simulink model "full_system"  (R2023b)
settings: Solver=VariableStepAuto  StartTime=0.0  StopTime=Tend  RelTol=1e-3
undefined symbols (not defined in the file): A, Af, B, beta_off_deg, beta_on_deg, C, Cd, control_case, D, f, g, G_rref, Ki_beta, Ki_r, Kp_beta, Kp_r, m, Mz_max, Mz_min, rho, rw, tf1, theta_front, Tmax_wheel, Tmin_wheel, tr
libraries: slpidlib x2
settings Model: Creator=GLORIA  LastModifiedBy=joseg
settings OptimizationCC: ReuseModelBlockBuffer=off

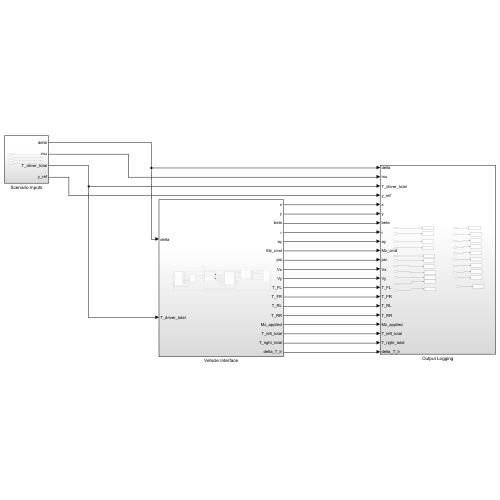
[thumbnail: Simulink's stored preview of the top-level diagram]
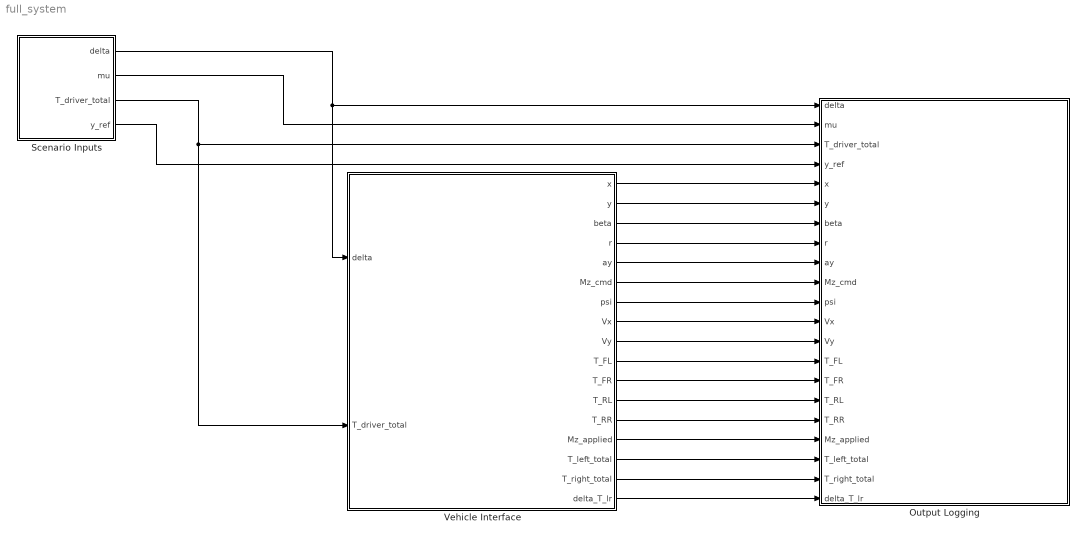
== system full_system ==
  Output Logging : Subsystem
  Scenario Inputs : Subsystem
  Vehicle Interface : Subsystem
  wires:
  Scenario Inputs/1(delta) -> Vehicle Interface/1(delta), Output Logging/1(delta)
  Scenario Inputs/2(mu) -> Output Logging/2(mu)
  Scenario Inputs/4(y_ref) -> Output Logging/4(y_ref)
  Vehicle Interface/1(x) -> Output Logging/5(x)
  Vehicle Interface/2(y) -> Output Logging/6(y)
  Vehicle Interface/3(beta) -> Output Logging/7(beta)
  Vehicle Interface/4(r) -> Output Logging/8(r)
  Vehicle Interface/5(ay) -> Output Logging/9(ay)
  Vehicle Interface/6(Mz_cmd) -> Output Logging/10(Mz_cmd)
  Vehicle Interface/7(psi) -> Output Logging/11(psi)
  Vehicle Interface/8(Vx) -> Output Logging/12(Vx)
  Vehicle Interface/9(Vy) -> Output Logging/13(Vy)
  Vehicle Interface/10(T_FL) -> Output Logging/14(T_FL)
  Vehicle Interface/11(T_FR) -> Output Logging/15(T_FR)
  Vehicle Interface/12(T_RL) -> Output Logging/16(T_RL)
  Vehicle Interface/13(T_RR) -> Output Logging/17(T_RR)
  Scenario Inputs/3(T_driver_total) -> Vehicle Interface/2(T_driver_total), Output Logging/3(T_driver_total)
  Vehicle Interface/14(Mz_applied) -> Output Logging/18(Mz_applied)
  Vehicle Interface/15(T_left_total) -> Output Logging/19(T_left_total)
  Vehicle Interface/16(T_right_total) -> Output Logging/20(T_right_total)
  Vehicle Interface/17(delta_T_lr) -> Output Logging/21(delta_T_lr)

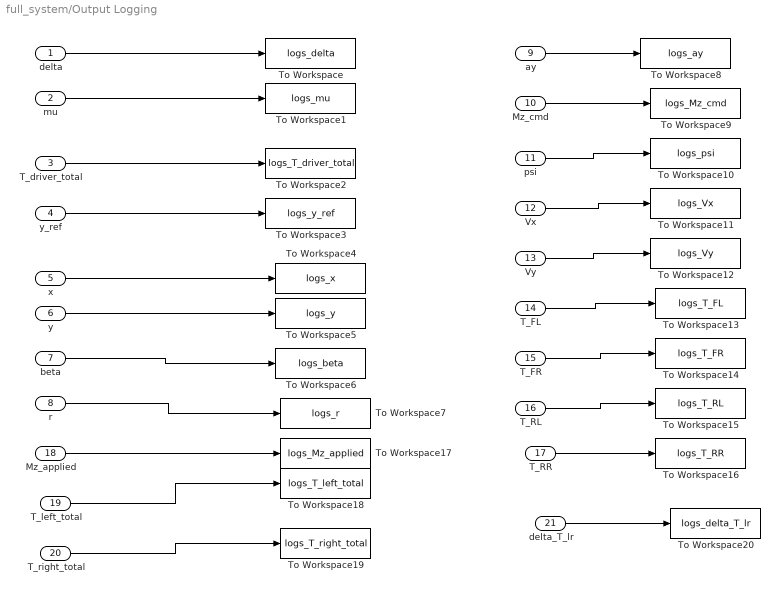
== system full_system/Output Logging ==
  delta : Inport
  mu : Inport  Port=2
  T_driver_total : Inport  Port=3
  y_ref : Inport  Port=4
  x : Inport  Port=5
  y : Inport  Port=6
  beta : Inport  Port=7
  r : Inport  Port=8
  ay : Inport  Port=9
  Mz_cmd : Inport  Port=10
  psi : Inport  Port=11
  Vx : Inport  Port=12
  Vy : Inport  Port=13
  T_FL : Inport  Port=14
  T_FR : Inport  Port=15
  T_RL : Inport  Port=16
  T_RR : Inport  Port=17
  Mz_applied : Inport  Port=18
  T_left_total : Inport  Port=19
  T_right_total : Inport  Port=20
  delta_T_lr : Inport  Port=21
  To Workspace : ToWorkspace  VariableName=logs_delta  SaveFormat=Timeseries  SampleTime=-1
  To Workspace1 : ToWorkspace  VariableName=logs_mu  SaveFormat=Timeseries  SampleTime=-1
  To Workspace10 : ToWorkspace  VariableName=logs_psi  SaveFormat=Timeseries  SampleTime=-1
  To Workspace11 : ToWorkspace  VariableName=logs_Vx  SaveFormat=Timeseries  SampleTime=-1
  To Workspace12 : ToWorkspace  VariableName=logs_Vy  SaveFormat=Timeseries  SampleTime=-1
  To Workspace13 : ToWorkspace  VariableName=logs_T_FL  SaveFormat=Timeseries  SampleTime=-1
  To Workspace14 : ToWorkspace  VariableName=logs_T_FR  SaveFormat=Timeseries  SampleTime=-1
  To Workspace15 : ToWorkspace  VariableName=logs_T_RL  SaveFormat=Timeseries  SampleTime=-1
  To Workspace16 : ToWorkspace  VariableName=logs_T_RR  SaveFormat=Timeseries  SampleTime=-1
  To Workspace17 : ToWorkspace  VariableName=logs_Mz_applied  SaveFormat=Timeseries  SampleTime=-1
  To Workspace18 : ToWorkspace  VariableName=logs_T_left_total  SaveFormat=Timeseries  SampleTime=-1
  To Workspace19 : ToWorkspace  VariableName=logs_T_right_total  SaveFormat=Timeseries  SampleTime=-1
  To Workspace2 : ToWorkspace  VariableName=logs_T_driver_total  SaveFormat=Timeseries  SampleTime=-1
  To Workspace20 : ToWorkspace  VariableName=logs_delta_T_lr  SaveFormat=Timeseries  SampleTime=-1
  To Workspace3 : ToWorkspace  VariableName=logs_y_ref  SaveFormat=Timeseries  SampleTime=-1
  To Workspace4 : ToWorkspace  VariableName=logs_x  SaveFormat=Timeseries  SampleTime=-1
  To Workspace5 : ToWorkspace  VariableName=logs_y  SaveFormat=Timeseries  SampleTime=-1
  To Workspace6 : ToWorkspace  VariableName=logs_beta  SaveFormat=Timeseries  SampleTime=-1
  To Workspace7 : ToWorkspace  VariableName=logs_r  SaveFormat=Timeseries  SampleTime=-1
  To Workspace8 : ToWorkspace  VariableName=logs_ay  SaveFormat=Timeseries  SampleTime=-1
  To Workspace9 : ToWorkspace  VariableName=logs_Mz_cmd  SaveFormat=Timeseries  SampleTime=-1
  wires:
  delta/1 -> To Workspace/1
  mu/1 -> To Workspace1/1
  T_driver_total/1 -> To Workspace2/1
  y_ref/1 -> To Workspace3/1
  x/1 -> To Workspace4/1
  y/1 -> To Workspace5/1
  beta/1 -> To Workspace6/1
  r/1 -> To Workspace7/1
  ay/1 -> To Workspace8/1
  Mz_cmd/1 -> To Workspace9/1
  psi/1 -> To Workspace10/1
  Vx/1 -> To Workspace11/1
  Vy/1 -> To Workspace12/1
  T_FL/1 -> To Workspace13/1
  T_FR/1 -> To Workspace14/1
  T_RL/1 -> To Workspace15/1
  T_RR/1 -> To Workspace16/1
  Mz_applied/1 -> To Workspace17/1
  delta_T_lr/1 -> To Workspace20/1
  T_left_total/1 -> To Workspace18/1
  T_right_total/1 -> To Workspace19/1

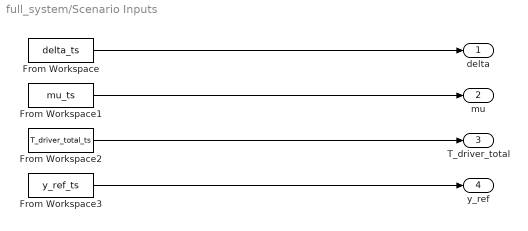
== system full_system/Scenario Inputs ==
  From Workspace : FromWorkspace  VariableName=delta_ts
  From Workspace1 : FromWorkspace  VariableName=mu_ts
  From Workspace2 : FromWorkspace  VariableName=T_driver_total_ts
  From Workspace3 : FromWorkspace  VariableName=y_ref_ts
  delta : Outport
  mu : Outport  Port=2
  T_driver_total : Outport  Port=3
  y_ref : Outport  Port=4
  wires:
  From Workspace/1 -> delta/1
  From Workspace1/1 -> mu/1
  From Workspace2/1 -> T_driver_total/1
  From Workspace3/1 -> y_ref/1

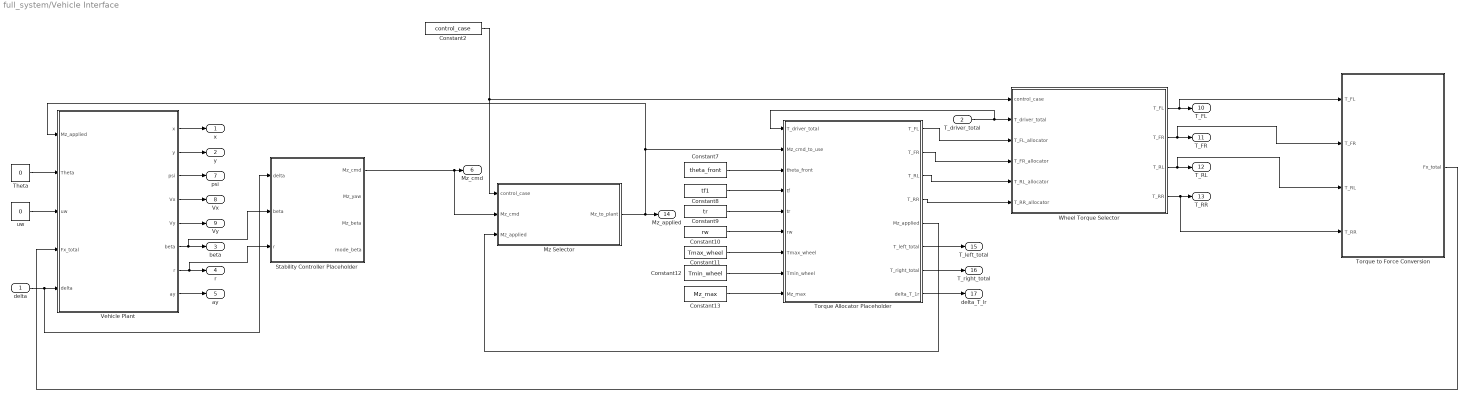
== system full_system/Vehicle Interface ==
  delta : Inport
  T_driver_total : Inport  Port=2
  Constant10 : Constant  Value=rw
  Constant11 : Constant  Value=Tmax_wheel
  Constant12 : Constant  Value=Tmin_wheel
  Constant13 : Constant  Value=Mz_max
  Constant2 : Constant  Value=control_case
  Constant7 : Constant  Value=theta_front
  Constant8 : Constant  Value=tf1
  Constant9 : Constant  Value=tr
  Mz Selector : Subsystem
  Stability Controller Placeholder : Subsystem
  Theta : Constant  Value=0
  Torque Allocator Placeholder : Subsystem
  Torque to Force Conversion : Subsystem
  Vehicle Plant : Subsystem
  Wheel Torque Selector : Subsystem
  uw : Constant  Value=0
  x : Outport
  y : Outport  Port=2
  beta : Outport  Port=3
  r : Outport  Port=4
  ay : Outport  Port=5
  Mz_cmd : Outport  Port=6
  psi : Outport  Port=7
  Vx : Outport  Port=8
  Vy : Outport  Port=9
  T_FL : Outport  Port=10
  T_FR : Outport  Port=11
  T_RL : Outport  Port=12
  T_RR : Outport  Port=13
  Mz_applied : Outport  Port=14
  T_left_total : Outport  Port=15
  T_right_total : Outport  Port=16
  delta_T_lr : Outport  Port=17
  wires:
  Theta/1 -> Vehicle Plant/2(Theta)
  uw/1 -> Vehicle Plant/3(uw)
  Vehicle Plant/1(x) -> x/1
  Vehicle Plant/2(y) -> y/1
  Vehicle Plant/3(psi) -> psi/1
  Vehicle Plant/4(Vx) -> Vx/1
  Vehicle Plant/5(Vy) -> Vy/1
  Vehicle Plant/6(beta) -> beta/1, Stability Controller Placeholder/2(beta)
  Vehicle Plant/7(r) -> r/1, Stability Controller Placeholder/3(r)
  Vehicle Plant/8(ay) -> ay/1
  T_driver_total/1 -> Torque Allocator Placeholder/1(T_driver_total), Wheel Torque Selector/2(T_driver_total)
  Torque to Force Conversion/1(Fx_total) -> Vehicle Plant/4(Fx_total)
  delta/1 -> Vehicle Plant/5(delta), Stability Controller Placeholder/1(delta)
  Stability Controller Placeholder/1(Mz_cmd) -> Mz Selector/2(Mz_cmd), Mz_cmd/1
  Mz Selector/1(Mz_to_plant) -> Mz_applied/1, Torque Allocator Placeholder/2(Mz_cmd_to_use), Vehicle Plant/1(Mz_applied)
  Wheel Torque Selector/1(T_FL) -> T_FL/1, Torque to Force Conversion/1(T_FL)
  Wheel Torque Selector/2(T_FR) -> Torque to Force Conversion/2(T_FR), T_FR/1
  Wheel Torque Selector/3(T_RL) -> T_RL/1, Torque to Force Conversion/3(T_RL)
  Wheel Torque Selector/4(T_RR) -> Torque to Force Conversion/4(T_RR), T_RR/1
  Torque Allocator Placeholder/1(T_FL) -> Wheel Torque Selector/3(T_FL_allocator)
  Torque Allocator Placeholder/2(T_FR) -> Wheel Torque Selector/4(T_FR_allocator)
  Torque Allocator Placeholder/3(T_RL) -> Wheel Torque Selector/5(T_RL_allocator)
  Torque Allocator Placeholder/4(T_RR) -> Wheel Torque Selector/6(T_RR_allocator)
  Torque Allocator Placeholder/5(Mz_applied) -> Mz Selector/3(Mz_applied)
  Constant2/1 -> Mz Selector/1(control_case), Wheel Torque Selector/1(control_case)
  Torque Allocator Placeholder/6(T_left_total) -> T_left_total/1
  Torque Allocator Placeholder/8(delta_T_1r) -> delta_T_lr/1
  Torque Allocator Placeholder/7(T_right_total) -> T_right_total/1
  Constant7/1 -> Torque Allocator Placeholder/3(theta_front)
  Constant8/1 -> Torque Allocator Placeholder/4(tf)
  Constant9/1 -> Torque Allocator Placeholder/5(tr)
  Constant10/1 -> Torque Allocator Placeholder/6(rw)
  Constant11/1 -> Torque Allocator Placeholder/7(Tmax_wheel)
  Constant12/1 -> Torque Allocator Placeholder/8(Tmin_wheel)
  Constant13/1 -> Torque Allocator Placeholder/9(Mz_max)

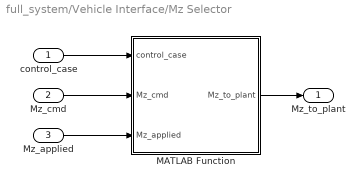
== system full_system/Vehicle Interface/Mz Selector ==
  control_case : Inport
  Mz_cmd : Inport  Port=2
  Mz_applied : Inport  Port=3
  MATLAB Function : MATLAB Function  TreatAsAtomicUnit=on
  Mz_to_plant : Outport
  wires:
  MATLAB Function/1(Mz_to_plant) -> Mz_to_plant/1
  Mz_cmd/1 -> MATLAB Function/2(Mz_cmd)
  Mz_applied/1 -> MATLAB Function/3(Mz_applied)
  control_case/1 -> MATLAB Function/1(control_case)

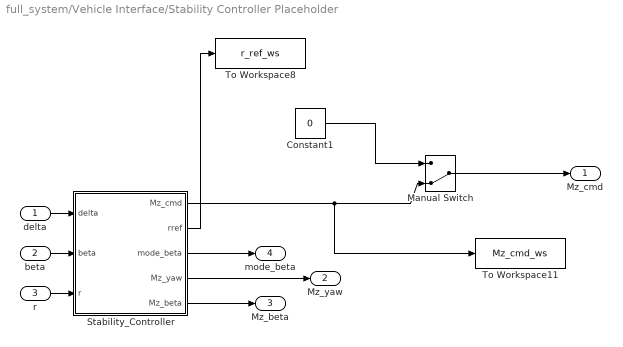
== system full_system/Vehicle Interface/Stability Controller Placeholder ==
  delta : Inport
  beta : Inport  Port=2
  r : Inport  Port=3
  Constant1 : Constant  Value=0
  Manual Switch : ManualSwitch  CurrentSetting=0
  Stability_Controller : Subsystem
  To Workspace11 : ToWorkspace  VariableName=Mz_cmd_ws  SaveFormat=Structure With Time  SampleTime=-1
      settings: Save2DSignal=2-D array (concatenate along first dimension)
  To Workspace8 : ToWorkspace  VariableName=r_ref_ws  SaveFormat=Structure With Time  SampleTime=-1
      settings: Save2DSignal=2-D array (concatenate along first dimension)
  Mz_cmd : Outport
  Mz_yaw : Outport  Port=2
  Mz_beta : Outport  Port=3
  mode_beta : Outport  Port=4
  wires:
  Stability_Controller/1(Mz_cmd) -> To Workspace11/1, Manual Switch/2
  Stability_Controller/2(rref) -> To Workspace8/1
  Constant1/1 -> Manual Switch/1
  delta/1 -> Stability_Controller/1(delta)
  beta/1 -> Stability_Controller/2(beta)
  r/1 -> Stability_Controller/3(r)
  Stability_Controller/3(mode_beta) -> mode_beta/1
  Manual Switch/1 -> Mz_cmd/1
  Stability_Controller/5(Mz_beta) -> Mz_beta/1
  Stability_Controller/4(Mz_yaw) -> Mz_yaw/1

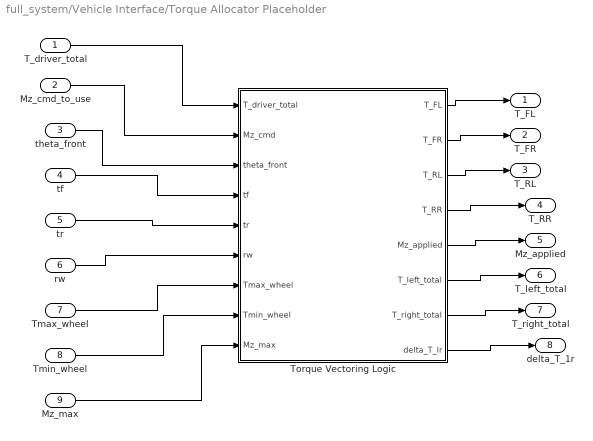
== system full_system/Vehicle Interface/Torque Allocator Placeholder ==
  T_driver_total : Inport
  Mz_cmd_to_use : Inport  Port=2
  theta_front : Inport  Port=3
  tf : Inport  Port=4
  tr : Inport  Port=5
  rw : Inport  Port=6
  Tmax_wheel : Inport  Port=7
  Tmin_wheel : Inport  Port=8
  Mz_max : Inport  Port=9
  Torque Vectoring Logic : MATLAB Function  TreatAsAtomicUnit=on
  T_FL : Outport
  T_FR : Outport  Port=2
  T_RL : Outport  Port=3
  T_RR : Outport  Port=4
  Mz_applied : Outport  Port=5
  T_left_total : Outport  Port=6
  T_right_total : Outport  Port=7
  delta_T_1r : Outport  Port=8
  wires:
  theta_front/1 -> Torque Vectoring Logic/3(theta_front)
  Tmax_wheel/1 -> Torque Vectoring Logic/7(Tmax_wheel)
  tr/1 -> Torque Vectoring Logic/5(tr)
  Mz_cmd_to_use/1 -> Torque Vectoring Logic/2(Mz_cmd)
  Tmin_wheel/1 -> Torque Vectoring Logic/8(Tmin_wheel)
  Mz_max/1 -> Torque Vectoring Logic/9(Mz_max)
  tf/1 -> Torque Vectoring Logic/4(tf)
  rw/1 -> Torque Vectoring Logic/6(rw)
  Torque Vectoring Logic/1(T_FL) -> T_FL/1
  Torque Vectoring Logic/2(T_FR) -> T_FR/1
  Torque Vectoring Logic/3(T_RL) -> T_RL/1
  Torque Vectoring Logic/4(T_RR) -> T_RR/1
  Torque Vectoring Logic/5(Mz_applied) -> Mz_applied/1
  Torque Vectoring Logic/6(T_left_total) -> T_left_total/1
  Torque Vectoring Logic/7(T_right_total) -> T_right_total/1
  Torque Vectoring Logic/8(delta_T_lr) -> delta_T_1r/1
  T_driver_total/1 -> Torque Vectoring Logic/1(T_driver_total)

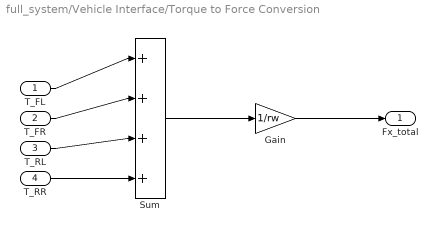
== system full_system/Vehicle Interface/Torque to Force Conversion ==
  T_FL : Inport
  T_FR : Inport  Port=2
  T_RL : Inport  Port=3
  T_RR : Inport  Port=4
  Gain : Gain  Gain=1/rw
  Sum : Sum  Inputs=|++++
  Fx_total : Outport
  wires:
  Gain/1 -> Fx_total/1
  T_FL/1 -> Sum/1
  T_FR/1 -> Sum/2
  T_RL/1 -> Sum/3
  T_RR/1 -> Sum/4
  Sum/1 -> Gain/1

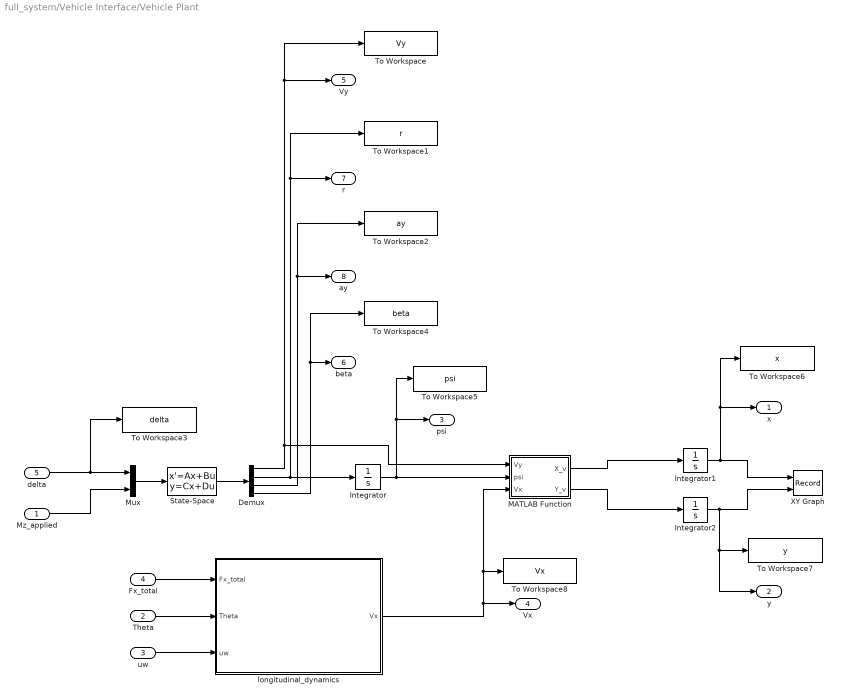
== system full_system/Vehicle Interface/Vehicle Plant ==
  Mz_applied : Inport
  Theta : Inport  Port=2
  uw : Inport  Port=3
  Fx_total : Inport  Port=4
  delta : Inport  Port=5
  Demux : Demux
  Integrator : Integrator
  Integrator1 : Integrator
  Integrator2 : Integrator
  MATLAB Function : MATLAB Function  TreatAsAtomicUnit=on
  Mux : Mux  Inputs=2
  State-Space : StateSpace  A=A  B=B  C=C  D=D  InitialCondition=[0;0]
  To Workspace : ToWorkspace  VariableName=Vy  SampleTime=-1
      settings: Save2DSignal=2-D array (concatenate along first dimension)
  To Workspace1 : ToWorkspace  VariableName=r  SampleTime=-1
      settings: Save2DSignal=2-D array (concatenate along first dimension)
  To Workspace2 : ToWorkspace  VariableName=ay  SampleTime=-1
      settings: Save2DSignal=2-D array (concatenate along first dimension)
  To Workspace3 : ToWorkspace  VariableName=delta  SampleTime=-1
      settings: Save2DSignal=2-D array (concatenate along first dimension)
  To Workspace4 : ToWorkspace  VariableName=beta  SampleTime=-1
      settings: Save2DSignal=2-D array (concatenate along first dimension)
  To Workspace5 : ToWorkspace  VariableName=psi  SampleTime=-1
      settings: Save2DSignal=2-D array (concatenate along first dimension)
  To Workspace6 : ToWorkspace  VariableName=x  SampleTime=-1
      settings: Save2DSignal=2-D array (concatenate along first dimension)
  To Workspace7 : ToWorkspace  VariableName=y  SampleTime=-1
      settings: Save2DSignal=2-D array (concatenate along first dimension)
  To Workspace8 : ToWorkspace  VariableName=Vx  SampleTime=-1
      settings: Save2DSignal=2-D array (concatenate along first dimension)
  XY Graph : Record  FileSettingsInternal="{\"entries\":[{\"content\":{\"excelSettings\":{\"content\":{},\"type\":\"Streamout.ExcelSettings\"}},\"type\":\"Streamout.FileSettingStorage\",\"uuid\":\"\"}],\"packageUris\":[\"http:\\/\\/schema.mathworks.com\\/mf0\\/streamout_blocks\\/R2020a\"],\"version\":\"1.0\"}"  Layout=[1 1]  SignalsInternal="{\"entries\":[{\"content\":{\"signals\":[{\"content\":{\"blockPath\":[],\"dimensions\":[1],\"domain\":\"\",\"lineColor\":\"#ff6929\",\"port\":1,\"signalID\":1,\"signalName\":\"Integrator1\"},\"type\":\"RecordBlkView.Signal\",\"uuid\":\"\"},{\"content\":{\"blockPath\":[],\"dimensions\":[1],\"domain\":\"\",\"lineColor\":\"#139fff\",\"plots\":[ 1 ],\"port\":2,\"signalID\":2,\"signalName\":\"Integrator2\"},\"type\":\"RecordBlkView.Signal\",\"uuid\":\"\"}]},\"type\":\"RecordBlkView.InputSignals\",\"uuid\":\"\"}],\"packageUris\":[\"http:\\/\\/schema.mathworks.com\\/mf0\\/streamout_blocks\\/R2020a\"],\"version\":\"1.0\"}"  VisualizationBindings="{\"xyplotplugin\":{\"info\":[{\"series\":[{\"bindingParametersList\":[{\"parameter\":\"Y-Axis\",\"signalID\":2,\"signalName\":\"Integrator2\"}],\"seriesID\":0}],\"subplotID\":1}]}}"  CompatibilityTag=XY
  longitudinal_dynamics : Subsystem
  x : Outport
  y : Outport  Port=2
  psi : Outport  Port=3
  Vx : Outport  Port=4
  Vy : Outport  Port=5
  beta : Outport  Port=6
  r : Outport  Port=7
  ay : Outport  Port=8
  wires:
  Integrator/1 -> psi/1, To Workspace5/1, MATLAB Function/2(psi)
  Demux/3 -> To Workspace2/1, ay/1
  Demux/4 -> To Workspace4/1, beta/1
  Integrator2/1 -> y/1, To Workspace7/1, XY Graph/2
  Integrator1/1 -> x/1, To Workspace6/1, XY Graph/1
  Demux/1 -> To Workspace/1, Vy/1, MATLAB Function/1(Vy)
  Theta/1 -> longitudinal_dynamics/2(Theta)
  MATLAB Function/2(Y_v) -> Integrator2/1
  Mux/1 -> State-Space/1
  MATLAB Function/1(X_v) -> Integrator1/1
  longitudinal_dynamics/1(Vx) -> MATLAB Function/3(Vx), To Workspace8/1, Vx/1
  State-Space/1 -> Demux/1
  uw/1 -> longitudinal_dynamics/3(uw)
  Mz_applied/1 -> Mux/2
  Demux/2 -> To Workspace1/1, r/1, Integrator/1
  Fx_total/1 -> longitudinal_dynamics/1(Fx_total)
  delta/1 -> Mux/1, To Workspace3/1

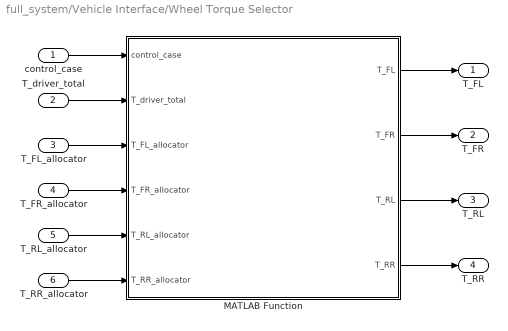
== system full_system/Vehicle Interface/Wheel Torque Selector ==
  control_case : Inport
  T_driver_total : Inport  Port=2
  T_FL_allocator : Inport  Port=3
  T_FR_allocator : Inport  Port=4
  T_RL_allocator : Inport  Port=5
  T_RR_allocator : Inport  Port=6
  MATLAB Function : MATLAB Function  TreatAsAtomicUnit=on
  T_FL : Outport
  T_FR : Outport  Port=2
  T_RL : Outport  Port=3
  T_RR : Outport  Port=4
  wires:
  MATLAB Function/1(T_FL) -> T_FL/1
  MATLAB Function/2(T_FR) -> T_FR/1
  MATLAB Function/3(T_RL) -> T_RL/1
  MATLAB Function/4(T_RR) -> T_RR/1
  control_case/1 -> MATLAB Function/1(control_case)
  T_driver_total/1 -> MATLAB Function/2(T_driver_total)
  T_FL_allocator/1 -> MATLAB Function/3(T_FL_allocator)
  T_RL_allocator/1 -> MATLAB Function/5(T_RL_allocator)
  T_FR_allocator/1 -> MATLAB Function/4(T_FR_allocator)
  T_RR_allocator/1 -> MATLAB Function/6(T_RR_allocator)

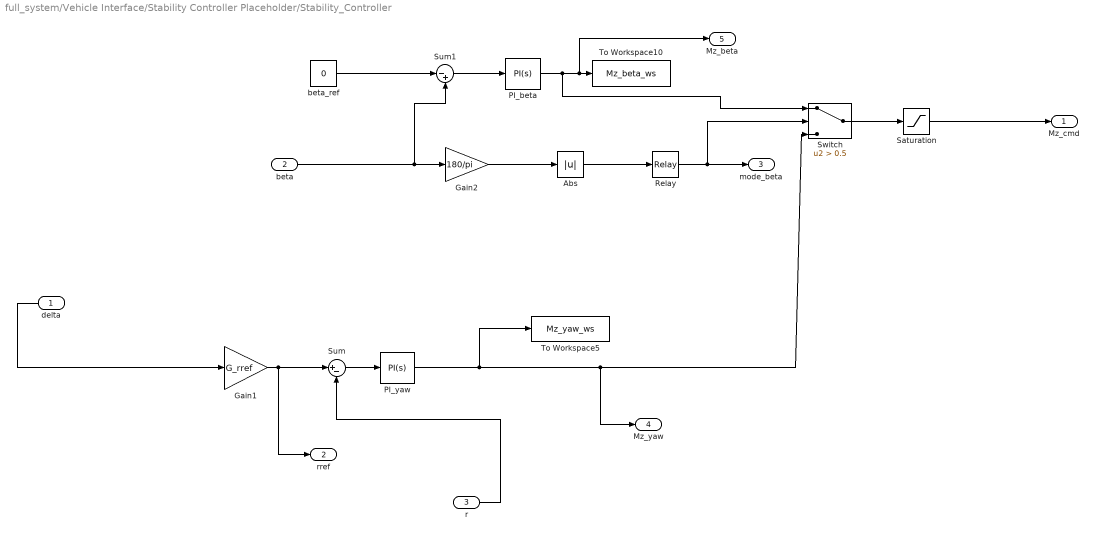
== system full_system/Vehicle Interface/Stability Controller Placeholder/Stability_Controller ==
  delta : Inport
  beta : Inport  Port=2
  r : Inport  Port=3
  Abs : Abs  SaturateOnIntegerOverflow=off
  Gain1 : Gain  Gain=G_rref
  Gain2 : Gain  Gain=180/pi
  PI_beta : slpidlib/PID Controller  Controller=PI  Form=Parallel  TimeDomain=Continuous-time  UseExternalTs=off  SampleTime=-1  IntegratorMethod=Forward Euler  FilterMethod=Forward Euler  ControllerParametersSource=internal  P=Kp_beta  I=Ki_beta  UseKiTs=off  D=0  N=100  UseFilter=on  TunerSelectOption=Transfer Function Based (PID Tuner App)  InitialConditionSource=internal  InitialConditionForIntegrator=0  InitialConditionForFilter=0  DifferentiatorICPrevScaledInput=0  ExternalReset=none  TrackingMode=off  Kt=1  LimitOutput=off  SatLimitsSource=internal  UpperSaturationLimit=inf  LowerSaturationLimit=-inf  LinearizeAsGain=on  AntiWindupMode=none  Kb=1  LimitIntegrator=off  UpperIntegratorSaturationLimit=inf  LowerIntegratorSaturationLimit=-inf  POutMin=[]  POutMax=[]  IOutMin=[]  IOutMax=[]  DOutMin=[]  DOutMax=[]  NOutMin=[]  NOutMax=[]  SumOutMin=[]  SumOutMax=[]  SaturationOutMin=[]  SaturationOutMax=[]  PParamMin=[]  PParamMax=[]  IParamMin=[]  IParamMax=[]  DParamMin=[]  DParamMax=[]  NParamMin=[]  NParamMax=[]  KbParamMin=[]  KbParamMax=[]  KtParamMin=[]  KtParamMax=[]  KbOutMin=[]  KbOutMax=[]  KtOutMin=[]  KtOutMax=[]  IntegratorOutMin=[]  IntegratorOutMax=[]  FilterOutMin=[]  FilterOutMax=[]  SumI1OutMin=[]  SumI1OutMax=[]  SumI2OutMin=[]  SumI2OutMax=[]  SumI3OutMin=[]  SumI3OutMax=[]  SumI4OutMin=[]  SumI4OutMax=[]  SumDOutMin=[]  SumDOutMax=[]  DifferentiatorOutMin=[]  DifferentiatorOutMax=[]  FilterDiffOutCoefMin=[]  FilterDiffOutCoefMax=[]  ReciprocalOutMin=[]  ReciprocalOutMax=[]  SumDenOutMin=[]  SumDenOutMax=[]  SumNumOutMin=[]  SumNumOutMax=[]  DivideOutMin=[]  DivideOutMax=[]  UdiffTsProdOutMin=[]  UdiffTsProdOutMax=[]  NTsProdOutMin=[]  NTsProdOutMax=[]  UintegralTsProdOutMin=[]  UintegralTsProdOutMax=[]  UngainTsProdOutMin=[]  UngainTsProdOutMax=[]  ClampingZeroOutDataTypeStr=Inherit: Inherit via back propagation  ClampingZeroOutMin=[]  ClampingZeroOutMax=[]  FilterDenConstantOutDataTypeStr=Inherit: Inherit via back propagation  FilterDenConstantOutMin=[]  FilterDenConstantOutMax=[]  PCopyOutDataTypeStr=Inherit: Inherit via back propagation  PCopyOutMin=[]  PCopyOutMax=[]  NCopyOutDataTypeStr=Inherit: Inherit via back propagation  NCopyOutMin=[]  NCopyOutMax=[]  IntegratorContinuousStateAttributes=''  IntegratorStateMustResolveToSignalObject=off  IntegratorRTWStateStorageClass=Auto  FilterContinuousStateAttributes=''  FilterStateMustResolveToSignalObject=off  FilterRTWStateStorageClass=Auto  ParallelPVariant=InternalParameters  IdealPVariant=Disabled  IVariant=InternalParameters  DVariant=Disabled  IntegratorVariant=Continuous  SatVariant=Disabled  AWVariant=Passthrough  PCopyVariant=Disabled  TRVariant=Disabled  FdbkBlocksVariant=Forward  IdealPFdbkVariant=Disabled  SatFdbkVariant=Disabled  DerivativeFilterVariant=Disabled  NVariant=Disabled  NCopyVariant=Disabled_SignalSpec  FilterICVariant=Disabled  IntegratorICVariant=InternalICs  ExternalResetVariant=Disabled  TRSumVariant=Passthrough  SumFdbkVariant=Disabled  SumVariant=Sum_PI  TsampFilterVariant=InternalTs  TsampNgainVariant=Passthrough  TsampIntegralVariant=Disabled_SignalSpec  ExternalSaturationOutDataTypeStr=Inherit: Same as second input
  PI_yaw : slpidlib/PID Controller  Controller=PI  Form=Parallel  TimeDomain=Continuous-time  UseExternalTs=off  SampleTime=-1  IntegratorMethod=Forward Euler  FilterMethod=Forward Euler  ControllerParametersSource=internal  P=Kp_r  I=Ki_r  UseKiTs=off  D=0  N=100  UseFilter=on  TunerSelectOption=Transfer Function Based (PID Tuner App)  InitialConditionSource=internal  InitialConditionForIntegrator=0  InitialConditionForFilter=0  DifferentiatorICPrevScaledInput=0  ExternalReset=none  TrackingMode=off  Kt=1  LimitOutput=off  SatLimitsSource=internal  UpperSaturationLimit=inf  LowerSaturationLimit=-inf  LinearizeAsGain=on  AntiWindupMode=none  Kb=1  LimitIntegrator=off  UpperIntegratorSaturationLimit=inf  LowerIntegratorSaturationLimit=-inf  POutMin=[]  POutMax=[]  IOutMin=[]  IOutMax=[]  DOutMin=[]  DOutMax=[]  NOutMin=[]  NOutMax=[]  SumOutMin=[]  SumOutMax=[]  SaturationOutMin=[]  SaturationOutMax=[]  PParamMin=[]  PParamMax=[]  IParamMin=[]  IParamMax=[]  DParamMin=[]  DParamMax=[]  NParamMin=[]  NParamMax=[]  KbParamMin=[]  KbParamMax=[]  KtParamMin=[]  KtParamMax=[]  KbOutMin=[]  KbOutMax=[]  KtOutMin=[]  KtOutMax=[]  IntegratorOutMin=[]  IntegratorOutMax=[]  FilterOutMin=[]  FilterOutMax=[]  SumI1OutMin=[]  SumI1OutMax=[]  SumI2OutMin=[]  SumI2OutMax=[]  SumI3OutMin=[]  SumI3OutMax=[]  SumI4OutMin=[]  SumI4OutMax=[]  SumDOutMin=[]  SumDOutMax=[]  DifferentiatorOutMin=[]  DifferentiatorOutMax=[]  FilterDiffOutCoefMin=[]  FilterDiffOutCoefMax=[]  ReciprocalOutMin=[]  ReciprocalOutMax=[]  SumDenOutMin=[]  SumDenOutMax=[]  SumNumOutMin=[]  SumNumOutMax=[]  DivideOutMin=[]  DivideOutMax=[]  UdiffTsProdOutMin=[]  UdiffTsProdOutMax=[]  NTsProdOutMin=[]  NTsProdOutMax=[]  UintegralTsProdOutMin=[]  UintegralTsProdOutMax=[]  UngainTsProdOutMin=[]  UngainTsProdOutMax=[]  ClampingZeroOutDataTypeStr=Inherit: Inherit via back propagation  ClampingZeroOutMin=[]  ClampingZeroOutMax=[]  FilterDenConstantOutDataTypeStr=Inherit: Inherit via back propagation  FilterDenConstantOutMin=[]  FilterDenConstantOutMax=[]  PCopyOutDataTypeStr=Inherit: Inherit via back propagation  PCopyOutMin=[]  PCopyOutMax=[]  NCopyOutDataTypeStr=Inherit: Inherit via back propagation  NCopyOutMin=[]  NCopyOutMax=[]  IntegratorContinuousStateAttributes=''  IntegratorStateMustResolveToSignalObject=off  IntegratorRTWStateStorageClass=Auto  FilterContinuousStateAttributes=''  FilterStateMustResolveToSignalObject=off  FilterRTWStateStorageClass=Auto  ParallelPVariant=InternalParameters  IdealPVariant=Disabled  IVariant=InternalParameters  DVariant=Disabled  IntegratorVariant=Continuous  SatVariant=Disabled  AWVariant=Passthrough  PCopyVariant=Disabled  TRVariant=Disabled  FdbkBlocksVariant=Forward  IdealPFdbkVariant=Disabled  SatFdbkVariant=Disabled  DerivativeFilterVariant=Disabled  NVariant=Disabled  NCopyVariant=Disabled_SignalSpec  FilterICVariant=Disabled  IntegratorICVariant=InternalICs  ExternalResetVariant=Disabled  TRSumVariant=Passthrough  SumFdbkVariant=Disabled  SumVariant=Sum_PI  TsampFilterVariant=InternalTs  TsampNgainVariant=Passthrough  TsampIntegralVariant=Disabled_SignalSpec  ExternalSaturationOutDataTypeStr=Inherit: Same as second input
  Relay : Relay  OnSwitchValue=beta_on_deg  OffSwitchValue=beta_off_deg
  Saturation : Saturate  UpperLimit=Mz_max  LowerLimit=Mz_min
  Sum : Sum  Inputs=|+-
  Sum1 : Sum  Inputs=|-+
  Switch : Switch  Criteria=u2 > Threshold  Threshold=0.5  SaturateOnIntegerOverflow=off  InputSameDT=off
  To Workspace10 : ToWorkspace  VariableName=Mz_beta_ws  SaveFormat=Structure With Time  SampleTime=-1
      settings: Save2DSignal=2-D array (concatenate along first dimension)
  To Workspace5 : ToWorkspace  VariableName=Mz_yaw_ws  SaveFormat=Structure With Time  SampleTime=-1
      settings: Save2DSignal=2-D array (concatenate along first dimension)
  beta_ref : Constant  Value=0
  Mz_cmd : Outport
  rref : Outport  Port=2
  mode_beta : Outport  Port=3
  Mz_yaw : Outport  Port=4
  Mz_beta : Outport  Port=5
  wires:
  beta_ref/1 -> Sum1/1
  Abs/1 -> Relay/1
  PI_beta/1 -> Switch/1, Mz_beta/1, To Workspace10/1
  beta/1 -> Sum1/2, Gain2/1
  PI_yaw/1 -> To Workspace5/1, Mz_yaw/1, Switch/3
  Gain2/1 -> Abs/1
  Sum/1 -> PI_yaw/1
  Sum1/1 -> PI_beta/1
  Gain1/1 -> rref/1, Sum/1
  delta/1 -> Gain1/1
  r/1 -> Sum/2
  Switch/1 -> Saturation/1
  Saturation/1 -> Mz_cmd/1
  Relay/1 -> Switch/2, mode_beta/1

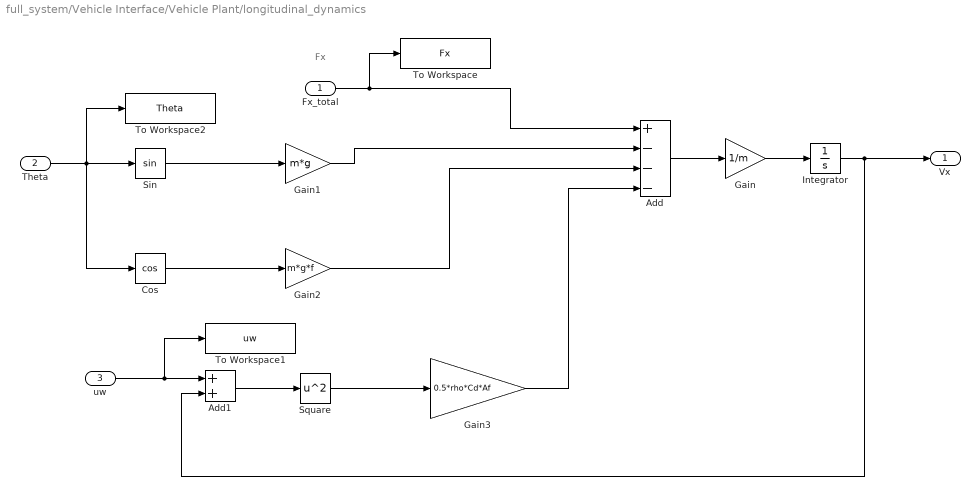
== system full_system/Vehicle Interface/Vehicle Plant/longitudinal_dynamics ==
  note: Fx
  Fx_total : Inport
  Theta : Inport  Port=2
  uw : Inport  Port=3
  Add : Sum  Inputs=+---
  Add1 : Sum
  Cos : Trigonometry  Operator=cos
  Gain : Gain  Gain=1/m
  Gain1 : Gain  Gain=m*g
  Gain2 : Gain  Gain=m*g*f
  Gain3 : Gain  Gain=0.5*rho*Cd*Af
  Integrator : Integrator  InitialCondition=16
  Sin : Trigonometry
  Square : Math  Operator=square
  To Workspace : ToWorkspace  VariableName=Fx  SampleTime=-1
      settings: Save2DSignal=2-D array (concatenate along first dimension)
  To Workspace1 : ToWorkspace  VariableName=uw  SampleTime=-1
      settings: Save2DSignal=2-D array (concatenate along first dimension)
  To Workspace2 : ToWorkspace  VariableName=Theta  SampleTime=-1
      settings: Save2DSignal=2-D array (concatenate along first dimension)
  Vx : Outport
  wires:
  Gain1/1 -> Add/2
  Add1/1 -> Square/1
  Add/1 -> Gain/1
  Gain2/1 -> Add/3
  Cos/1 -> Gain2/1
  Square/1 -> Gain3/1
  Gain/1 -> Integrator/1
  uw/1 -> To Workspace1/1, Add1/1
  Theta/1 -> To Workspace2/1, Cos/1, Sin/1
  Sin/1 -> Gain1/1
  Gain3/1 -> Add/4
  Fx_total/1 -> To Workspace/1, Add/1
  Integrator/1 -> Add1/2, Vx/1

== matlab function full_system/Vehicle Interface/Torque Allocator Placeholder/Torque Vectoring Logic ==
  data: T_driver_total input; T_FL output; Mz_cmd input; theta_front input; tf input; tr input; rw input; Tmax_wheel input; Tmin_wheel input; Mz_max input; T_FR output; T_RL output; T_RR output; Mz_applied output; T_left_total output; T_right_total output; delta_T_lr output
function [T_FL, T_FR, T_RL, T_RR, Mz_applied, T_left_total, T_right_total, delta_T_lr] = fcn(T_driver_total, Mz_cmd, theta_front, tf, tr, rw, Tmax_wheel, Tmin_wheel, Mz_max)

% Saturate requested yaw moment
if Mz_cmd > Mz_max
    Mz_cmd = Mz_max;
elseif Mz_cmd < -Mz_max
    Mz_cmd = -Mz_max;
end

% Nominal symmetric torque distribution
T_nom = T_driver_total / 4;

T_FL_nom = T_nom;
T_FR_nom = T_nom;
T_RL_nom = T_nom;
T_RR_nom = T_nom;

% Split yaw moment between front and rear axle
Mz_front = theta_front * Mz_cmd;
Mz_rear  = (1 - theta_front) * Mz_cmd;

% Convert yaw moment into left-right torque difference
dT_front = (Mz_front * rw) / tf;
dT_rear  = (Mz_rear  * rw) / tr;

% Positive Mz: more torque on right wheels, less on left wheels
T_FL = T_FL_nom - dT_front;
T_FR = T_FR_nom + dT_front;
T_RL = T_RL_nom - dT_rear;
T_RR = T_RR_nom + dT_rear;

% Wheel torque saturation
T_FL = min(max(T_FL, Tmin_wheel), Tmax_wheel);
T_FR = min(max(T_FR, Tmin_wheel), Tmax_wheel);
T_RL = min(max(T_RL, Tmin_wheel), Tmax_wheel);
T_RR = min(max(T_RR, Tmin_wheel), Tmax_wheel);

% Estimate actually generated yaw moment after saturation
Fx_FL = T_FL / rw;
Fx_FR = T_FR / rw;
Fx_RL = T_RL / rw;
Fx_RR = T_RR / rw;

Mz_front_applied = (Fx_FR - Fx_FL) * tf / 2;
Mz_rear_applied  = (Fx_RR - Fx_RL) * tr / 2;

Mz_applied = Mz_front_applied + Mz_rear_applied;

% Additional outputs for analysis and plots
T_left_total  = T_FL + T_RL;
T_right_total = T_FR + T_RR;
delta_T_lr    = T_right_total - T_left_total;

end

== matlab function full_system/Vehicle Interface/Vehicle Plant/MATLAB Function ==
  data: Vy input; X_v output; psi input; Vx input; Y_v output
function [X_v, Y_v] = fcn(Vy, psi, Vx)

X_v = Vx*cos(psi) - Vy*sin(psi);
Y_v = Vx*sin(psi) + Vy*cos(psi);

end

== matlab function full_system/Vehicle Interface/Mz Selector/MATLAB Function ==
  data: control_case input; Mz_to_plant output; Mz_cmd input; Mz_applied input
function Mz_to_plant = select_mz(control_case, Mz_cmd, Mz_applied)

if control_case == 0
    Mz_to_plant = 0;
elseif control_case == 1
    Mz_to_plant = Mz_cmd;
else
    Mz_to_plant = Mz_applied;
end

end

== matlab function full_system/Vehicle Interface/Wheel Torque Selector/MATLAB Function ==
  data: control_case input; T_FL output; T_driver_total input; T_FL_allocator input; T_FR_allocator input; T_RL_allocator input; T_RR_allocator input; T_FR output; T_RL output; T_RR output
function [T_FL, T_FR, T_RL, T_RR] = select_wheel_torques( ...
    control_case, T_driver_total, ...
    T_FL_allocator, T_FR_allocator, T_RL_allocator, T_RR_allocator)

if control_case == 2
    T_FL = T_FL_allocator;
    T_FR = T_FR_allocator;
    T_RL = T_RL_allocator;
    T_RR = T_RR_allocator;
else
    T_FL = T_driver_total / 4;
    T_FR = T_driver_total / 4;
    T_RL = T_driver_total / 4;
    T_RR = T_driver_total / 4;
end

end
